simulink model "Voltage_Vector_with_script_fianl"  (R2024b)
settings: Solver=FixedStepAuto  StartTime=0.0  StopTime=0.5  FixedStep=1e-5  RelTol=1e-3
model workspace (MAT data in the model file):
  Cap = 0.004
  FL = 0.025
  Indcut = 0.005
  Initial_Voltage = 125
  R_Load = 1000
  V_dc = 300
  Vd = 125
  Vl = 400
  c = 125
  cap = 7.07e-05
  f_o = 50
  f_s = 5000
libraries: spsIGBTDiodeLib x72, spsSeriesRLCBranchLib x48, spsMultimeterLib x9, spsRMSLib x7, spsThreePhaseBreakerLib x6, spsTHDLib x6, spsThreePhaseSeriesRLCLoadLib x4, spsGroundLib x3, spsCurrentMeasurementLib x2, spsDCVoltageSourceLib x2, spsThreePhaseVIMeasurementLib x2, slpidlib x1
(part 1 of 3)
settings Model: Creator=Ravinga  LastModifiedBy=Sampa
settings DataIOCC: ReturnWorkspaceOutputs=off

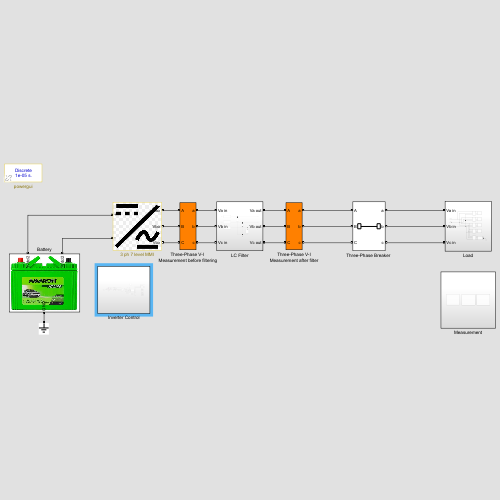
[thumbnail: Simulink's stored preview of the top-level diagram]
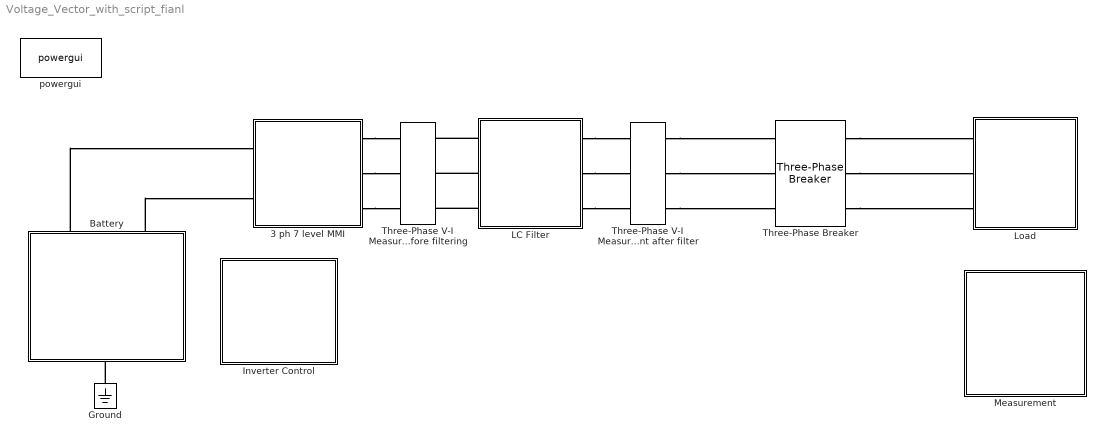
== system Voltage_Vector_with_script_fianl ==
  3 ph 7 level MMI : Subsystem
      mask Display: image('$imagefile'); % Use "Edit Image" on toolstrip to change.
  Battery : Subsystem
      settings: PortSchema="{\"entries\":[{\"content\":{\"sides\":[{\"content\":{},\"type\":\"ConnectorPlacement.EquallySpacedRectSide\",\"uuid\":\"8b3d1574-355a-4c35-8c5c-de7b51b3cb30\"},{\"content\":{\"side\":\"RIGHT\"},\"type\":\"ConnectorPlacement.EquallySpacedRectSide\",\"uuid\":\"59478119-0728-40d5-b667-b9fe531f9ab0\"},{\"content\":{\"connectorIds\":[\"LConn1\",\"LConn2\"],\"side\":\"TOP\"},\"type\":\"ConnectorPlacement.EquallySpacedRectSide\",\"uuid\":\"4590429d-f6cd-431e-b965-edb08c3a41e8\"},{\"content\":{\"connectorIds\":[\"RConn1\"],\"side\":\"BOTTOM\"},\"type\":\"ConnectorPlacement.EquallySpacedRectSide\",\"uuid\":\"66b38a99-a54a-47db-8935-0704255e048e\"}]},\"type\":\"ConnectorPlacement.EquallySpacedConnector\",\"uuid\":\"702254ea-54ff-4f66-b397-10c2b421dddc\"}],\"packageUris\":[\"http://schema.mathworks.com/mf0/Connector/R2020b\"],\"version\":\"1.0\"}"
      mask Display: image('12-v-amaron-battery.jpg');
  Ground : spsGroundLib/Ground  LConnTagsString=a
  Inverter Control : Subsystem
  LC Filter : Subsystem
  Load : Subsystem
  Measurement : Subsystem
  "Three-Phase Breaker " : spsThreePhaseBreakerLib/Three-Phase Breaker  InitialState=closed  SwitchA=on  SwitchB=on  SwitchC=on  SwitchTimes="[1/60  5/60]"  External=off  BreakerResistance=0.01  SnubberResistance=inf  SnubberCapacitance=inf  Measurements=None
  Three-Phase V-I Measurement after filter : spsThreePhaseVIMeasurementLib/Three-Phase V-I Measurement  VoltageMeasurement=phase-to-ground  SetLabelV=on  LabelV=Vabc_af  Vpu=off  VpuLL=off  CurrentMeasurement=yes  SetLabelI=on  LabelI=Iabc_af  Ipu=off  Pbase=100e6  Vbase=500e3  OutputType=Complex  PhasorSimulation=off  PSBequivalent=0
  Three-Phase V-I Measurement before filtering : spsThreePhaseVIMeasurementLib/Three-Phase V-I Measurement  VoltageMeasurement=phase-to-ground  SetLabelV=on  LabelV=Vabc_bf  Vpu=off  VpuLL=off  CurrentMeasurement=yes  SetLabelI=on  LabelI=Iabc_bf  Ipu=off  Pbase=100e6  Vbase=500e3  OutputType=Complex  PhasorSimulation=off  PSBequivalent=0
  powergui : spspowerguiLib/powergui  Priority=1  SimulationMode=Discrete  SampleTime=1e-5  frequency=60  Iterations=50  frequencyindice=0  Pbase=100e6  ErrMax=1e-4  UnitsV=kV  UnitsW=MW  buscounter=0  FunctionMessages=off  echomessages=off  EnableUseOfTLC=off  CurrentSourceSwitches=off  DisableSnubberDevices=off  DisableRonSwitches=off  DisableVfSwitches=off  DisplayEquations=off  AutomaticDiscreteSolvers=off  SolverType=Tustin/Backward Euler (TBE)  Interpol=off  ExternalGateDelay=off  methode=off  Ts=100  x0status=blocks  SPID=on  SwTol=0  HookPort=off  NonlinearTolerance=1e-4  nMaxIteration=100  ContinueOnMaxIteration=off  RestoreLinks=warning  ResistiveCurrentMeasurement=off  Frange=[0:2:500]  Ylog=off  Xlog=on  ShowGrid=off  save=off  variable=ZData  structure=0  ZoomFFT=off  StartTime=0.0  cycles=1  DisplayStyle=1  fundamental=60  FreqAxis=off  MaxFrequency=1000  frequencyindicesteady=1  RmsSteady=1  display=off
  connections:
  3 ph 7 level MMI/RConn1 -- Three-Phase V-I Measurement before filtering/LConn1
  3 ph 7 level MMI/RConn2 -- Three-Phase V-I Measurement before filtering/LConn2
  3 ph 7 level MMI/RConn3 -- Three-Phase V-I Measurement before filtering/LConn3
  "Three-Phase Breaker "/RConn1 -- Load/LConn1
  "Three-Phase Breaker "/RConn2 -- Load/LConn2
  "Three-Phase Breaker "/RConn3 -- Load/LConn3
  LC Filter/LConn1 -- Three-Phase V-I Measurement before filtering/RConn1
  LC Filter/LConn2 -- Three-Phase V-I Measurement before filtering/RConn2
  LC Filter/LConn3 -- Three-Phase V-I Measurement before filtering/RConn3
  LC Filter/RConn1 -- Three-Phase V-I Measurement after filter/LConn1
  LC Filter/RConn2 -- Three-Phase V-I Measurement after filter/LConn2
  LC Filter/RConn3 -- Three-Phase V-I Measurement after filter/LConn3
  Battery/LConn1 -- 3 ph 7 level MMI/LConn1
  Battery/LConn2 -- 3 ph 7 level MMI/LConn2
  Ground/LConn1 -- Battery/RConn1
  Three-Phase V-I Measurement after filter/RConn1 -- "Three-Phase Breaker "/LConn1
  Three-Phase V-I Measurement after filter/RConn2 -- "Three-Phase Breaker "/LConn2
  Three-Phase V-I Measurement after filter/RConn3 -- "Three-Phase Breaker "/LConn3

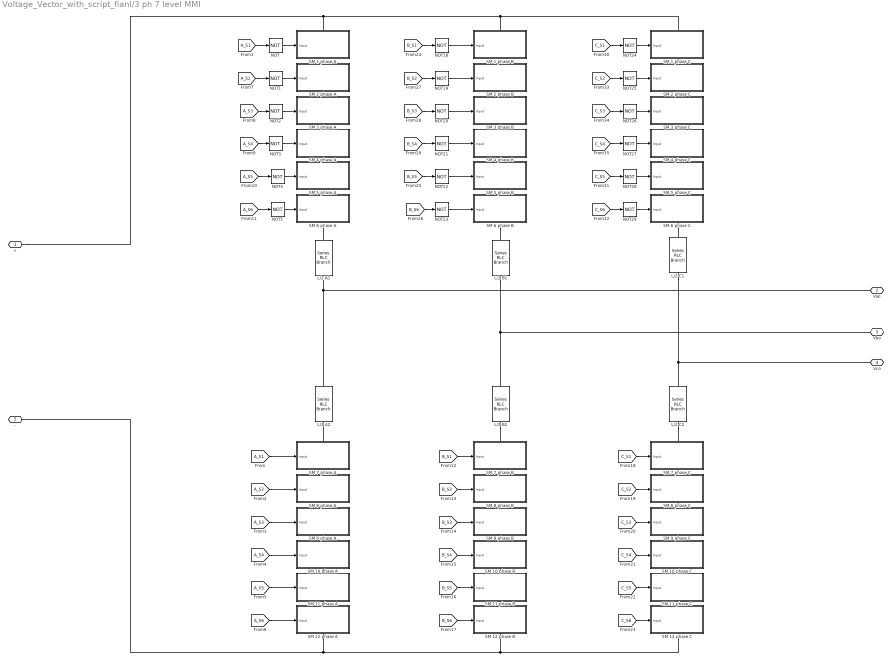
== system Voltage_Vector_with_script_fianl/3 ph 7 level MMI ==
  L/2 A1 : spsSeriesRLCBranchLib/Series RLC Branch  LConnTagsString=__new0  RConnTagsString=__new0  BranchType=L  Resistance=1  Inductance=Indcut  SetiL0=off  InitialCurrent=0  Capacitance=1e-6  Setx0=off  InitialVoltage=0  Measurements=Branch voltage and current
  L/2 A2 : spsSeriesRLCBranchLib/Series RLC Branch  LConnTagsString=__new0  RConnTagsString=__new0  BranchType=L  Resistance=1  Inductance=Indcut  SetiL0=off  InitialCurrent=0  Capacitance=1e-6  Setx0=off  InitialVoltage=0  Measurements=Branch voltage and current
  L/2 B1 : spsSeriesRLCBranchLib/Series RLC Branch  LConnTagsString=__new0  RConnTagsString=__new0  BranchType=L  Resistance=1  Inductance=Indcut  SetiL0=off  InitialCurrent=0  Capacitance=1e-6  Setx0=off  InitialVoltage=0  Measurements=Branch voltage and current
  L/2 B2 : spsSeriesRLCBranchLib/Series RLC Branch  LConnTagsString=__new0  RConnTagsString=__new0  BranchType=L  Resistance=1  Inductance=Indcut  SetiL0=off  InitialCurrent=0  Capacitance=1e-6  Setx0=off  InitialVoltage=0  Measurements=Branch voltage and current
  L/2 C1 : spsSeriesRLCBranchLib/Series RLC Branch  LConnTagsString=__new0  RConnTagsString=__new0  BranchType=L  Resistance=1  Inductance=Indcut  SetiL0=off  InitialCurrent=0  Capacitance=1e-6  Setx0=off  InitialVoltage=0  Measurements=Branch voltage and current
  L/2 C2 : spsSeriesRLCBranchLib/Series RLC Branch  LConnTagsString=__new0  RConnTagsString=__new0  BranchType=L  Resistance=1  Inductance=Indcut  SetiL0=off  InitialCurrent=0  Capacitance=1e-6  Setx0=off  InitialVoltage=0  Measurements=Branch voltage and current
  NOT{,1..5,18..29} (18 alike) : Logic  Operator=NOT  IconShape=distinctive  AllPortsSameDT=off  OutDataTypeStr=boolean
  SM 1 phase A : Subsystem
      settings: PortSchema="{\"entries\":[{\"content\":{\"sides\":[{\"content\":{\"connectorIds\":[\"In1\"]},\"type\":\"ConnectorPlacement.EquallySpacedRectSide\",\"uuid\":\"a2a6df29-5e25-4a5c-b62e-0f1ae4b64f0e\"},{\"content\":{\"connectorIds\":[],\"side\":\"RIGHT\"},\"type\":\"ConnectorPlacement.EquallySpacedRectSide\",\"uuid\":\"30b08227-6494-43ba-ab8b-c0acd0c21381\"},{\"content\":{\"connectorIds\":[\"LConn1\"],\"side\":\"TOP\"},\"type\":\"ConnectorPlacement.EquallySpacedRectSide\",\"uuid\":\"a6e05eb5-068d-4625-ba30-3a309ab3e04e\"},{\"content\":{\"connectorIds\":[\"RConn1\"],\"side\":\"BOTTOM\"},\"type\":\"ConnectorPlacement.EquallySpacedRectSide\",\"uuid\":\"593874a1-6541-4ba7-a8c9-20c2ddfecffb\"}]},\"type\":\"ConnectorPlacement.EquallySpacedConnector\",\"uuid\":\"7a0dd57a-dc4f-41ff-a1a4-3a20e1ff1320\"}],\"packageUris\":[\"http://schema.mathworks.com/mf0/Connector/R2020b\"],\"version\":\"1.0\"}"
  SM 1 phase B : Subsystem
      settings: PortSchema="{\"entries\":[{\"content\":{\"sides\":[{\"content\":{\"connectorIds\":[\"In1\"]},\"type\":\"ConnectorPlacement.EquallySpacedRectSide\",\"uuid\":\"a2a6df29-5e25-4a5c-b62e-0f1ae4b64f0e\"},{\"content\":{\"connectorIds\":[],\"side\":\"RIGHT\"},\"type\":\"ConnectorPlacement.EquallySpacedRectSide\",\"uuid\":\"30b08227-6494-43ba-ab8b-c0acd0c21381\"},{\"content\":{\"connectorIds\":[\"LConn1\"],\"side\":\"TOP\"},\"type\":\"ConnectorPlacement.EquallySpacedRectSide\",\"uuid\":\"a6e05eb5-068d-4625-ba30-3a309ab3e04e\"},{\"content\":{\"connectorIds\":[\"RConn1\"],\"side\":\"BOTTOM\"},\"type\":\"ConnectorPlacement.EquallySpacedRectSide\",\"uuid\":\"593874a1-6541-4ba7-a8c9-20c2ddfecffb\"}]},\"type\":\"ConnectorPlacement.EquallySpacedConnector\",\"uuid\":\"7a0dd57a-dc4f-41ff-a1a4-3a20e1ff1320\"}],\"packageUris\":[\"http://schema.mathworks.com/mf0/Connector/R2020b\"],\"version\":\"1.0\"}"
  SM 1 phase C : Subsystem
      settings: PortSchema="{\"entries\":[{\"content\":{\"sides\":[{\"content\":{\"connectorIds\":[\"In1\"]},\"type\":\"ConnectorPlacement.EquallySpacedRectSide\",\"uuid\":\"a2a6df29-5e25-4a5c-b62e-0f1ae4b64f0e\"},{\"content\":{\"connectorIds\":[],\"side\":\"RIGHT\"},\"type\":\"ConnectorPlacement.EquallySpacedRectSide\",\"uuid\":\"30b08227-6494-43ba-ab8b-c0acd0c21381\"},{\"content\":{\"connectorIds\":[\"LConn1\"],\"side\":\"TOP\"},\"type\":\"ConnectorPlacement.EquallySpacedRectSide\",\"uuid\":\"a6e05eb5-068d-4625-ba30-3a309ab3e04e\"},{\"content\":{\"connectorIds\":[\"RConn1\"],\"side\":\"BOTTOM\"},\"type\":\"ConnectorPlacement.EquallySpacedRectSide\",\"uuid\":\"593874a1-6541-4ba7-a8c9-20c2ddfecffb\"}]},\"type\":\"ConnectorPlacement.EquallySpacedConnector\",\"uuid\":\"7a0dd57a-dc4f-41ff-a1a4-3a20e1ff1320\"}],\"packageUris\":[\"http://schema.mathworks.com/mf0/Connector/R2020b\"],\"version\":\"1.0\"}"
  SM 10 phase A : Subsystem
      settings: PortSchema="{\"entries\":[{\"content\":{\"sides\":[{\"content\":{\"connectorIds\":[\"In1\"]},\"type\":\"ConnectorPlacement.EquallySpacedRectSide\",\"uuid\":\"a2a6df29-5e25-4a5c-b62e-0f1ae4b64f0e\"},{\"content\":{\"connectorIds\":[],\"side\":\"RIGHT\"},\"type\":\"ConnectorPlacement.EquallySpacedRectSide\",\"uuid\":\"30b08227-6494-43ba-ab8b-c0acd0c21381\"},{\"content\":{\"connectorIds\":[\"LConn1\"],\"side\":\"TOP\"},\"type\":\"ConnectorPlacement.EquallySpacedRectSide\",\"uuid\":\"a6e05eb5-068d-4625-ba30-3a309ab3e04e\"},{\"content\":{\"connectorIds\":[\"RConn1\"],\"side\":\"BOTTOM\"},\"type\":\"ConnectorPlacement.EquallySpacedRectSide\",\"uuid\":\"593874a1-6541-4ba7-a8c9-20c2ddfecffb\"}]},\"type\":\"ConnectorPlacement.EquallySpacedConnector\",\"uuid\":\"7a0dd57a-dc4f-41ff-a1a4-3a20e1ff1320\"}],\"packageUris\":[\"http://schema.mathworks.com/mf0/Connector/R2020b\"],\"version\":\"1.0\"}"
  SM 10 phase B : Subsystem
      settings: PortSchema="{\"entries\":[{\"content\":{\"sides\":[{\"content\":{\"connectorIds\":[\"In1\"]},\"type\":\"ConnectorPlacement.EquallySpacedRectSide\",\"uuid\":\"a2a6df29-5e25-4a5c-b62e-0f1ae4b64f0e\"},{\"content\":{\"connectorIds\":[],\"side\":\"RIGHT\"},\"type\":\"ConnectorPlacement.EquallySpacedRectSide\",\"uuid\":\"30b08227-6494-43ba-ab8b-c0acd0c21381\"},{\"content\":{\"connectorIds\":[\"LConn1\"],\"side\":\"TOP\"},\"type\":\"ConnectorPlacement.EquallySpacedRectSide\",\"uuid\":\"a6e05eb5-068d-4625-ba30-3a309ab3e04e\"},{\"content\":{\"connectorIds\":[\"RConn1\"],\"side\":\"BOTTOM\"},\"type\":\"ConnectorPlacement.EquallySpacedRectSide\",\"uuid\":\"593874a1-6541-4ba7-a8c9-20c2ddfecffb\"}]},\"type\":\"ConnectorPlacement.EquallySpacedConnector\",\"uuid\":\"7a0dd57a-dc4f-41ff-a1a4-3a20e1ff1320\"}],\"packageUris\":[\"http://schema.mathworks.com/mf0/Connector/R2020b\"],\"version\":\"1.0\"}"
  SM 10 phase C : Subsystem
      settings: PortSchema="{\"entries\":[{\"content\":{\"sides\":[{\"content\":{\"connectorIds\":[\"In1\"]},\"type\":\"ConnectorPlacement.EquallySpacedRectSide\",\"uuid\":\"a2a6df29-5e25-4a5c-b62e-0f1ae4b64f0e\"},{\"content\":{\"connectorIds\":[],\"side\":\"RIGHT\"},\"type\":\"ConnectorPlacement.EquallySpacedRectSide\",\"uuid\":\"30b08227-6494-43ba-ab8b-c0acd0c21381\"},{\"content\":{\"connectorIds\":[\"LConn1\"],\"side\":\"TOP\"},\"type\":\"ConnectorPlacement.EquallySpacedRectSide\",\"uuid\":\"a6e05eb5-068d-4625-ba30-3a309ab3e04e\"},{\"content\":{\"connectorIds\":[\"RConn1\"],\"side\":\"BOTTOM\"},\"type\":\"ConnectorPlacement.EquallySpacedRectSide\",\"uuid\":\"593874a1-6541-4ba7-a8c9-20c2ddfecffb\"}]},\"type\":\"ConnectorPlacement.EquallySpacedConnector\",\"uuid\":\"7a0dd57a-dc4f-41ff-a1a4-3a20e1ff1320\"}],\"packageUris\":[\"http://schema.mathworks.com/mf0/Connector/R2020b\"],\"version\":\"1.0\"}"
  SM 11 phase A : Subsystem
      settings: PortSchema="{\"entries\":[{\"content\":{\"sides\":[{\"content\":{\"connectorIds\":[\"In1\"]},\"type\":\"ConnectorPlacement.EquallySpacedRectSide\",\"uuid\":\"a2a6df29-5e25-4a5c-b62e-0f1ae4b64f0e\"},{\"content\":{\"connectorIds\":[],\"side\":\"RIGHT\"},\"type\":\"ConnectorPlacement.EquallySpacedRectSide\",\"uuid\":\"30b08227-6494-43ba-ab8b-c0acd0c21381\"},{\"content\":{\"connectorIds\":[\"LConn1\"],\"side\":\"TOP\"},\"type\":\"ConnectorPlacement.EquallySpacedRectSide\",\"uuid\":\"a6e05eb5-068d-4625-ba30-3a309ab3e04e\"},{\"content\":{\"connectorIds\":[\"RConn1\"],\"side\":\"BOTTOM\"},\"type\":\"ConnectorPlacement.EquallySpacedRectSide\",\"uuid\":\"593874a1-6541-4ba7-a8c9-20c2ddfecffb\"}]},\"type\":\"ConnectorPlacement.EquallySpacedConnector\",\"uuid\":\"7a0dd57a-dc4f-41ff-a1a4-3a20e1ff1320\"}],\"packageUris\":[\"http://schema.mathworks.com/mf0/Connector/R2020b\"],\"version\":\"1.0\"}"
  SM 11 phase B : Subsystem
      settings: PortSchema="{\"entries\":[{\"content\":{\"sides\":[{\"content\":{\"connectorIds\":[\"In1\"]},\"type\":\"ConnectorPlacement.EquallySpacedRectSide\",\"uuid\":\"a2a6df29-5e25-4a5c-b62e-0f1ae4b64f0e\"},{\"content\":{\"connectorIds\":[],\"side\":\"RIGHT\"},\"type\":\"ConnectorPlacement.EquallySpacedRectSide\",\"uuid\":\"30b08227-6494-43ba-ab8b-c0acd0c21381\"},{\"content\":{\"connectorIds\":[\"LConn1\"],\"side\":\"TOP\"},\"type\":\"ConnectorPlacement.EquallySpacedRectSide\",\"uuid\":\"a6e05eb5-068d-4625-ba30-3a309ab3e04e\"},{\"content\":{\"connectorIds\":[\"RConn1\"],\"side\":\"BOTTOM\"},\"type\":\"ConnectorPlacement.EquallySpacedRectSide\",\"uuid\":\"593874a1-6541-4ba7-a8c9-20c2ddfecffb\"}]},\"type\":\"ConnectorPlacement.EquallySpacedConnector\",\"uuid\":\"7a0dd57a-dc4f-41ff-a1a4-3a20e1ff1320\"}],\"packageUris\":[\"http://schema.mathworks.com/mf0/Connector/R2020b\"],\"version\":\"1.0\"}"
  SM 11 phase C : Subsystem
      settings: PortSchema="{\"entries\":[{\"content\":{\"sides\":[{\"content\":{\"connectorIds\":[\"In1\"]},\"type\":\"ConnectorPlacement.EquallySpacedRectSide\",\"uuid\":\"a2a6df29-5e25-4a5c-b62e-0f1ae4b64f0e\"},{\"content\":{\"connectorIds\":[],\"side\":\"RIGHT\"},\"type\":\"ConnectorPlacement.EquallySpacedRectSide\",\"uuid\":\"30b08227-6494-43ba-ab8b-c0acd0c21381\"},{\"content\":{\"connectorIds\":[\"LConn1\"],\"side\":\"TOP\"},\"type\":\"ConnectorPlacement.EquallySpacedRectSide\",\"uuid\":\"a6e05eb5-068d-4625-ba30-3a309ab3e04e\"},{\"content\":{\"connectorIds\":[\"RConn1\"],\"side\":\"BOTTOM\"},\"type\":\"ConnectorPlacement.EquallySpacedRectSide\",\"uuid\":\"593874a1-6541-4ba7-a8c9-20c2ddfecffb\"}]},\"type\":\"ConnectorPlacement.EquallySpacedConnector\",\"uuid\":\"7a0dd57a-dc4f-41ff-a1a4-3a20e1ff1320\"}],\"packageUris\":[\"http://schema.mathworks.com/mf0/Connector/R2020b\"],\"version\":\"1.0\"}"
  SM 12 phase A : Subsystem
      settings: PortSchema="{\"entries\":[{\"content\":{\"sides\":[{\"content\":{\"connectorIds\":[\"In1\"]},\"type\":\"ConnectorPlacement.EquallySpacedRectSide\",\"uuid\":\"a2a6df29-5e25-4a5c-b62e-0f1ae4b64f0e\"},{\"content\":{\"connectorIds\":[],\"side\":\"RIGHT\"},\"type\":\"ConnectorPlacement.EquallySpacedRectSide\",\"uuid\":\"30b08227-6494-43ba-ab8b-c0acd0c21381\"},{\"content\":{\"connectorIds\":[\"LConn1\"],\"side\":\"TOP\"},\"type\":\"ConnectorPlacement.EquallySpacedRectSide\",\"uuid\":\"a6e05eb5-068d-4625-ba30-3a309ab3e04e\"},{\"content\":{\"connectorIds\":[\"RConn1\"],\"side\":\"BOTTOM\"},\"type\":\"ConnectorPlacement.EquallySpacedRectSide\",\"uuid\":\"593874a1-6541-4ba7-a8c9-20c2ddfecffb\"}]},\"type\":\"ConnectorPlacement.EquallySpacedConnector\",\"uuid\":\"7a0dd57a-dc4f-41ff-a1a4-3a20e1ff1320\"}],\"packageUris\":[\"http://schema.mathworks.com/mf0/Connector/R2020b\"],\"version\":\"1.0\"}"
  SM 12 phase B : Subsystem
      settings: PortSchema="{\"entries\":[{\"content\":{\"sides\":[{\"content\":{\"connectorIds\":[\"In1\"]},\"type\":\"ConnectorPlacement.EquallySpacedRectSide\",\"uuid\":\"a2a6df29-5e25-4a5c-b62e-0f1ae4b64f0e\"},{\"content\":{\"connectorIds\":[],\"side\":\"RIGHT\"},\"type\":\"ConnectorPlacement.EquallySpacedRectSide\",\"uuid\":\"30b08227-6494-43ba-ab8b-c0acd0c21381\"},{\"content\":{\"connectorIds\":[\"LConn1\"],\"side\":\"TOP\"},\"type\":\"ConnectorPlacement.EquallySpacedRectSide\",\"uuid\":\"a6e05eb5-068d-4625-ba30-3a309ab3e04e\"},{\"content\":{\"connectorIds\":[\"RConn1\"],\"side\":\"BOTTOM\"},\"type\":\"ConnectorPlacement.EquallySpacedRectSide\",\"uuid\":\"593874a1-6541-4ba7-a8c9-20c2ddfecffb\"}]},\"type\":\"ConnectorPlacement.EquallySpacedConnector\",\"uuid\":\"7a0dd57a-dc4f-41ff-a1a4-3a20e1ff1320\"}],\"packageUris\":[\"http://schema.mathworks.com/mf0/Connector/R2020b\"],\"version\":\"1.0\"}"
  SM 12 phase C : Subsystem
      settings: PortSchema="{\"entries\":[{\"content\":{\"sides\":[{\"content\":{\"connectorIds\":[\"In1\"]},\"type\":\"ConnectorPlacement.EquallySpacedRectSide\",\"uuid\":\"a2a6df29-5e25-4a5c-b62e-0f1ae4b64f0e\"},{\"content\":{\"connectorIds\":[],\"side\":\"RIGHT\"},\"type\":\"ConnectorPlacement.EquallySpacedRectSide\",\"uuid\":\"30b08227-6494-43ba-ab8b-c0acd0c21381\"},{\"content\":{\"connectorIds\":[\"LConn1\"],\"side\":\"TOP\"},\"type\":\"ConnectorPlacement.EquallySpacedRectSide\",\"uuid\":\"a6e05eb5-068d-4625-ba30-3a309ab3e04e\"},{\"content\":{\"connectorIds\":[\"RConn1\"],\"side\":\"BOTTOM\"},\"type\":\"ConnectorPlacement.EquallySpacedRectSide\",\"uuid\":\"593874a1-6541-4ba7-a8c9-20c2ddfecffb\"}]},\"type\":\"ConnectorPlacement.EquallySpacedConnector\",\"uuid\":\"7a0dd57a-dc4f-41ff-a1a4-3a20e1ff1320\"}],\"packageUris\":[\"http://schema.mathworks.com/mf0/Connector/R2020b\"],\"version\":\"1.0\"}"
  SM 2 phase A : Subsystem
      settings: PortSchema="{\"entries\":[{\"content\":{\"sides\":[{\"content\":{\"connectorIds\":[\"In1\"]},\"type\":\"ConnectorPlacement.EquallySpacedRectSide\",\"uuid\":\"a2a6df29-5e25-4a5c-b62e-0f1ae4b64f0e\"},{\"content\":{\"connectorIds\":[],\"side\":\"RIGHT\"},\"type\":\"ConnectorPlacement.EquallySpacedRectSide\",\"uuid\":\"30b08227-6494-43ba-ab8b-c0acd0c21381\"},{\"content\":{\"connectorIds\":[\"LConn1\"],\"side\":\"TOP\"},\"type\":\"ConnectorPlacement.EquallySpacedRectSide\",\"uuid\":\"a6e05eb5-068d-4625-ba30-3a309ab3e04e\"},{\"content\":{\"connectorIds\":[\"RConn1\"],\"side\":\"BOTTOM\"},\"type\":\"ConnectorPlacement.EquallySpacedRectSide\",\"uuid\":\"593874a1-6541-4ba7-a8c9-20c2ddfecffb\"}]},\"type\":\"ConnectorPlacement.EquallySpacedConnector\",\"uuid\":\"7a0dd57a-dc4f-41ff-a1a4-3a20e1ff1320\"}],\"packageUris\":[\"http://schema.mathworks.com/mf0/Connector/R2020b\"],\"version\":\"1.0\"}"
  SM 2 phase B : Subsystem
      settings: PortSchema="{\"entries\":[{\"content\":{\"sides\":[{\"content\":{\"connectorIds\":[\"In1\"]},\"type\":\"ConnectorPlacement.EquallySpacedRectSide\",\"uuid\":\"a2a6df29-5e25-4a5c-b62e-0f1ae4b64f0e\"},{\"content\":{\"connectorIds\":[],\"side\":\"RIGHT\"},\"type\":\"ConnectorPlacement.EquallySpacedRectSide\",\"uuid\":\"30b08227-6494-43ba-ab8b-c0acd0c21381\"},{\"content\":{\"connectorIds\":[\"LConn1\"],\"side\":\"TOP\"},\"type\":\"ConnectorPlacement.EquallySpacedRectSide\",\"uuid\":\"a6e05eb5-068d-4625-ba30-3a309ab3e04e\"},{\"content\":{\"connectorIds\":[\"RConn1\"],\"side\":\"BOTTOM\"},\"type\":\"ConnectorPlacement.EquallySpacedRectSide\",\"uuid\":\"593874a1-6541-4ba7-a8c9-20c2ddfecffb\"}]},\"type\":\"ConnectorPlacement.EquallySpacedConnector\",\"uuid\":\"7a0dd57a-dc4f-41ff-a1a4-3a20e1ff1320\"}],\"packageUris\":[\"http://schema.mathworks.com/mf0/Connector/R2020b\"],\"version\":\"1.0\"}"
  SM 2 phase C : Subsystem
      settings: PortSchema="{\"entries\":[{\"content\":{\"sides\":[{\"content\":{\"connectorIds\":[\"In1\"]},\"type\":\"ConnectorPlacement.EquallySpacedRectSide\",\"uuid\":\"a2a6df29-5e25-4a5c-b62e-0f1ae4b64f0e\"},{\"content\":{\"connectorIds\":[],\"side\":\"RIGHT\"},\"type\":\"ConnectorPlacement.EquallySpacedRectSide\",\"uuid\":\"30b08227-6494-43ba-ab8b-c0acd0c21381\"},{\"content\":{\"connectorIds\":[\"LConn1\"],\"side\":\"TOP\"},\"type\":\"ConnectorPlacement.EquallySpacedRectSide\",\"uuid\":\"a6e05eb5-068d-4625-ba30-3a309ab3e04e\"},{\"content\":{\"connectorIds\":[\"RConn1\"],\"side\":\"BOTTOM\"},\"type\":\"ConnectorPlacement.EquallySpacedRectSide\",\"uuid\":\"593874a1-6541-4ba7-a8c9-20c2ddfecffb\"}]},\"type\":\"ConnectorPlacement.EquallySpacedConnector\",\"uuid\":\"7a0dd57a-dc4f-41ff-a1a4-3a20e1ff1320\"}],\"packageUris\":[\"http://schema.mathworks.com/mf0/Connector/R2020b\"],\"version\":\"1.0\"}"
  SM 3 phase A : Subsystem
      settings: PortSchema="{\"entries\":[{\"content\":{\"sides\":[{\"content\":{\"connectorIds\":[\"In1\"]},\"type\":\"ConnectorPlacement.EquallySpacedRectSide\",\"uuid\":\"a2a6df29-5e25-4a5c-b62e-0f1ae4b64f0e\"},{\"content\":{\"connectorIds\":[],\"side\":\"RIGHT\"},\"type\":\"ConnectorPlacement.EquallySpacedRectSide\",\"uuid\":\"30b08227-6494-43ba-ab8b-c0acd0c21381\"},{\"content\":{\"connectorIds\":[\"LConn1\"],\"side\":\"TOP\"},\"type\":\"ConnectorPlacement.EquallySpacedRectSide\",\"uuid\":\"a6e05eb5-068d-4625-ba30-3a309ab3e04e\"},{\"content\":{\"connectorIds\":[\"RConn1\"],\"side\":\"BOTTOM\"},\"type\":\"ConnectorPlacement.EquallySpacedRectSide\",\"uuid\":\"593874a1-6541-4ba7-a8c9-20c2ddfecffb\"}]},\"type\":\"ConnectorPlacement.EquallySpacedConnector\",\"uuid\":\"7a0dd57a-dc4f-41ff-a1a4-3a20e1ff1320\"}],\"packageUris\":[\"http://schema.mathworks.com/mf0/Connector/R2020b\"],\"version\":\"1.0\"}"
  SM 3 phase B : Subsystem
      settings: PortSchema="{\"entries\":[{\"content\":{\"sides\":[{\"content\":{\"connectorIds\":[\"In1\"]},\"type\":\"ConnectorPlacement.EquallySpacedRectSide\",\"uuid\":\"a2a6df29-5e25-4a5c-b62e-0f1ae4b64f0e\"},{\"content\":{\"connectorIds\":[],\"side\":\"RIGHT\"},\"type\":\"ConnectorPlacement.EquallySpacedRectSide\",\"uuid\":\"30b08227-6494-43ba-ab8b-c0acd0c21381\"},{\"content\":{\"connectorIds\":[\"LConn1\"],\"side\":\"TOP\"},\"type\":\"ConnectorPlacement.EquallySpacedRectSide\",\"uuid\":\"a6e05eb5-068d-4625-ba30-3a309ab3e04e\"},{\"content\":{\"connectorIds\":[\"RConn1\"],\"side\":\"BOTTOM\"},\"type\":\"ConnectorPlacement.EquallySpacedRectSide\",\"uuid\":\"593874a1-6541-4ba7-a8c9-20c2ddfecffb\"}]},\"type\":\"ConnectorPlacement.EquallySpacedConnector\",\"uuid\":\"7a0dd57a-dc4f-41ff-a1a4-3a20e1ff1320\"}],\"packageUris\":[\"http://schema.mathworks.com/mf0/Connector/R2020b\"],\"version\":\"1.0\"}"
  SM 3 phase C : Subsystem
      settings: PortSchema="{\"entries\":[{\"content\":{\"sides\":[{\"content\":{\"connectorIds\":[\"In1\"]},\"type\":\"ConnectorPlacement.EquallySpacedRectSide\",\"uuid\":\"a2a6df29-5e25-4a5c-b62e-0f1ae4b64f0e\"},{\"content\":{\"connectorIds\":[],\"side\":\"RIGHT\"},\"type\":\"ConnectorPlacement.EquallySpacedRectSide\",\"uuid\":\"30b08227-6494-43ba-ab8b-c0acd0c21381\"},{\"content\":{\"connectorIds\":[\"LConn1\"],\"side\":\"TOP\"},\"type\":\"ConnectorPlacement.EquallySpacedRectSide\",\"uuid\":\"a6e05eb5-068d-4625-ba30-3a309ab3e04e\"},{\"content\":{\"connectorIds\":[\"RConn1\"],\"side\":\"BOTTOM\"},\"type\":\"ConnectorPlacement.EquallySpacedRectSide\",\"uuid\":\"593874a1-6541-4ba7-a8c9-20c2ddfecffb\"}]},\"type\":\"ConnectorPlacement.EquallySpacedConnector\",\"uuid\":\"7a0dd57a-dc4f-41ff-a1a4-3a20e1ff1320\"}],\"packageUris\":[\"http://schema.mathworks.com/mf0/Connector/R2020b\"],\"version\":\"1.0\"}"
  SM 4 phase A : Subsystem
      settings: PortSchema="{\"entries\":[{\"content\":{\"sides\":[{\"content\":{\"connectorIds\":[\"In1\"]},\"type\":\"ConnectorPlacement.EquallySpacedRectSide\",\"uuid\":\"a2a6df29-5e25-4a5c-b62e-0f1ae4b64f0e\"},{\"content\":{\"connectorIds\":[],\"side\":\"RIGHT\"},\"type\":\"ConnectorPlacement.EquallySpacedRectSide\",\"uuid\":\"30b08227-6494-43ba-ab8b-c0acd0c21381\"},{\"content\":{\"connectorIds\":[\"LConn1\"],\"side\":\"TOP\"},\"type\":\"ConnectorPlacement.EquallySpacedRectSide\",\"uuid\":\"a6e05eb5-068d-4625-ba30-3a309ab3e04e\"},{\"content\":{\"connectorIds\":[\"RConn1\"],\"side\":\"BOTTOM\"},\"type\":\"ConnectorPlacement.EquallySpacedRectSide\",\"uuid\":\"593874a1-6541-4ba7-a8c9-20c2ddfecffb\"}]},\"type\":\"ConnectorPlacement.EquallySpacedConnector\",\"uuid\":\"7a0dd57a-dc4f-41ff-a1a4-3a20e1ff1320\"}],\"packageUris\":[\"http://schema.mathworks.com/mf0/Connector/R2020b\"],\"version\":\"1.0\"}"
  SM 4 phase B : Subsystem
      settings: PortSchema="{\"entries\":[{\"content\":{\"sides\":[{\"content\":{\"connectorIds\":[\"In1\"]},\"type\":\"ConnectorPlacement.EquallySpacedRectSide\",\"uuid\":\"a2a6df29-5e25-4a5c-b62e-0f1ae4b64f0e\"},{\"content\":{\"connectorIds\":[],\"side\":\"RIGHT\"},\"type\":\"ConnectorPlacement.EquallySpacedRectSide\",\"uuid\":\"30b08227-6494-43ba-ab8b-c0acd0c21381\"},{\"content\":{\"connectorIds\":[\"LConn1\"],\"side\":\"TOP\"},\"type\":\"ConnectorPlacement.EquallySpacedRectSide\",\"uuid\":\"a6e05eb5-068d-4625-ba30-3a309ab3e04e\"},{\"content\":{\"connectorIds\":[\"RConn1\"],\"side\":\"BOTTOM\"},\"type\":\"ConnectorPlacement.EquallySpacedRectSide\",\"uuid\":\"593874a1-6541-4ba7-a8c9-20c2ddfecffb\"}]},\"type\":\"ConnectorPlacement.EquallySpacedConnector\",\"uuid\":\"7a0dd57a-dc4f-41ff-a1a4-3a20e1ff1320\"}],\"packageUris\":[\"http://schema.mathworks.com/mf0/Connector/R2020b\"],\"version\":\"1.0\"}"
  SM 4 phase C : Subsystem
      settings: PortSchema="{\"entries\":[{\"content\":{\"sides\":[{\"content\":{\"connectorIds\":[\"In1\"]},\"type\":\"ConnectorPlacement.EquallySpacedRectSide\",\"uuid\":\"a2a6df29-5e25-4a5c-b62e-0f1ae4b64f0e\"},{\"content\":{\"connectorIds\":[],\"side\":\"RIGHT\"},\"type\":\"ConnectorPlacement.EquallySpacedRectSide\",\"uuid\":\"30b08227-6494-43ba-ab8b-c0acd0c21381\"},{\"content\":{\"connectorIds\":[\"LConn1\"],\"side\":\"TOP\"},\"type\":\"ConnectorPlacement.EquallySpacedRectSide\",\"uuid\":\"a6e05eb5-068d-4625-ba30-3a309ab3e04e\"},{\"content\":{\"connectorIds\":[\"RConn1\"],\"side\":\"BOTTOM\"},\"type\":\"ConnectorPlacement.EquallySpacedRectSide\",\"uuid\":\"593874a1-6541-4ba7-a8c9-20c2ddfecffb\"}]},\"type\":\"ConnectorPlacement.EquallySpacedConnector\",\"uuid\":\"7a0dd57a-dc4f-41ff-a1a4-3a20e1ff1320\"}],\"packageUris\":[\"http://schema.mathworks.com/mf0/Connector/R2020b\"],\"version\":\"1.0\"}"
  SM 5 phase A : Subsystem
      settings: PortSchema="{\"entries\":[{\"content\":{\"sides\":[{\"content\":{\"connectorIds\":[\"In1\"]},\"type\":\"ConnectorPlacement.EquallySpacedRectSide\",\"uuid\":\"a2a6df29-5e25-4a5c-b62e-0f1ae4b64f0e\"},{\"content\":{\"connectorIds\":[],\"side\":\"RIGHT\"},\"type\":\"ConnectorPlacement.EquallySpacedRectSide\",\"uuid\":\"30b08227-6494-43ba-ab8b-c0acd0c21381\"},{\"content\":{\"connectorIds\":[\"LConn1\"],\"side\":\"TOP\"},\"type\":\"ConnectorPlacement.EquallySpacedRectSide\",\"uuid\":\"a6e05eb5-068d-4625-ba30-3a309ab3e04e\"},{\"content\":{\"connectorIds\":[\"RConn1\"],\"side\":\"BOTTOM\"},\"type\":\"ConnectorPlacement.EquallySpacedRectSide\",\"uuid\":\"593874a1-6541-4ba7-a8c9-20c2ddfecffb\"}]},\"type\":\"ConnectorPlacement.EquallySpacedConnector\",\"uuid\":\"7a0dd57a-dc4f-41ff-a1a4-3a20e1ff1320\"}],\"packageUris\":[\"http://schema.mathworks.com/mf0/Connector/R2020b\"],\"version\":\"1.0\"}"
  SM 5 phase B : Subsystem
      settings: PortSchema="{\"entries\":[{\"content\":{\"sides\":[{\"content\":{\"connectorIds\":[\"In1\"]},\"type\":\"ConnectorPlacement.EquallySpacedRectSide\",\"uuid\":\"a2a6df29-5e25-4a5c-b62e-0f1ae4b64f0e\"},{\"content\":{\"connectorIds\":[],\"side\":\"RIGHT\"},\"type\":\"ConnectorPlacement.EquallySpacedRectSide\",\"uuid\":\"30b08227-6494-43ba-ab8b-c0acd0c21381\"},{\"content\":{\"connectorIds\":[\"LConn1\"],\"side\":\"TOP\"},\"type\":\"ConnectorPlacement.EquallySpacedRectSide\",\"uuid\":\"a6e05eb5-068d-4625-ba30-3a309ab3e04e\"},{\"content\":{\"connectorIds\":[\"RConn1\"],\"side\":\"BOTTOM\"},\"type\":\"ConnectorPlacement.EquallySpacedRectSide\",\"uuid\":\"593874a1-6541-4ba7-a8c9-20c2ddfecffb\"}]},\"type\":\"ConnectorPlacement.EquallySpacedConnector\",\"uuid\":\"7a0dd57a-dc4f-41ff-a1a4-3a20e1ff1320\"}],\"packageUris\":[\"http://schema.mathworks.com/mf0/Connector/R2020b\"],\"version\":\"1.0\"}"
  SM 5 phase C : Subsystem
      settings: PortSchema="{\"entries\":[{\"content\":{\"sides\":[{\"content\":{\"connectorIds\":[\"In1\"]},\"type\":\"ConnectorPlacement.EquallySpacedRectSide\",\"uuid\":\"a2a6df29-5e25-4a5c-b62e-0f1ae4b64f0e\"},{\"content\":{\"connectorIds\":[],\"side\":\"RIGHT\"},\"type\":\"ConnectorPlacement.EquallySpacedRectSide\",\"uuid\":\"30b08227-6494-43ba-ab8b-c0acd0c21381\"},{\"content\":{\"connectorIds\":[\"LConn1\"],\"side\":\"TOP\"},\"type\":\"ConnectorPlacement.EquallySpacedRectSide\",\"uuid\":\"a6e05eb5-068d-4625-ba30-3a309ab3e04e\"},{\"content\":{\"connectorIds\":[\"RConn1\"],\"side\":\"BOTTOM\"},\"type\":\"ConnectorPlacement.EquallySpacedRectSide\",\"uuid\":\"593874a1-6541-4ba7-a8c9-20c2ddfecffb\"}]},\"type\":\"ConnectorPlacement.EquallySpacedConnector\",\"uuid\":\"7a0dd57a-dc4f-41ff-a1a4-3a20e1ff1320\"}],\"packageUris\":[\"http://schema.mathworks.com/mf0/Connector/R2020b\"],\"version\":\"1.0\"}"
  SM 6 phase A : Subsystem
      settings: PortSchema="{\"entries\":[{\"content\":{\"sides\":[{\"content\":{\"connectorIds\":[\"In1\"]},\"type\":\"ConnectorPlacement.EquallySpacedRectSide\",\"uuid\":\"a2a6df29-5e25-4a5c-b62e-0f1ae4b64f0e\"},{\"content\":{\"connectorIds\":[],\"side\":\"RIGHT\"},\"type\":\"ConnectorPlacement.EquallySpacedRectSide\",\"uuid\":\"30b08227-6494-43ba-ab8b-c0acd0c21381\"},{\"content\":{\"connectorIds\":[\"LConn1\"],\"side\":\"TOP\"},\"type\":\"ConnectorPlacement.EquallySpacedRectSide\",\"uuid\":\"a6e05eb5-068d-4625-ba30-3a309ab3e04e\"},{\"content\":{\"connectorIds\":[\"RConn1\"],\"side\":\"BOTTOM\"},\"type\":\"ConnectorPlacement.EquallySpacedRectSide\",\"uuid\":\"593874a1-6541-4ba7-a8c9-20c2ddfecffb\"}]},\"type\":\"ConnectorPlacement.EquallySpacedConnector\",\"uuid\":\"7a0dd57a-dc4f-41ff-a1a4-3a20e1ff1320\"}],\"packageUris\":[\"http://schema.mathworks.com/mf0/Connector/R2020b\"],\"version\":\"1.0\"}"
  SM 6 phase B : Subsystem
      settings: PortSchema="{\"entries\":[{\"content\":{\"sides\":[{\"content\":{\"connectorIds\":[\"In1\"]},\"type\":\"ConnectorPlacement.EquallySpacedRectSide\",\"uuid\":\"a2a6df29-5e25-4a5c-b62e-0f1ae4b64f0e\"},{\"content\":{\"connectorIds\":[],\"side\":\"RIGHT\"},\"type\":\"ConnectorPlacement.EquallySpacedRectSide\",\"uuid\":\"30b08227-6494-43ba-ab8b-c0acd0c21381\"},{\"content\":{\"connectorIds\":[\"LConn1\"],\"side\":\"TOP\"},\"type\":\"ConnectorPlacement.EquallySpacedRectSide\",\"uuid\":\"a6e05eb5-068d-4625-ba30-3a309ab3e04e\"},{\"content\":{\"connectorIds\":[\"RConn1\"],\"side\":\"BOTTOM\"},\"type\":\"ConnectorPlacement.EquallySpacedRectSide\",\"uuid\":\"593874a1-6541-4ba7-a8c9-20c2ddfecffb\"}]},\"type\":\"ConnectorPlacement.EquallySpacedConnector\",\"uuid\":\"7a0dd57a-dc4f-41ff-a1a4-3a20e1ff1320\"}],\"packageUris\":[\"http://schema.mathworks.com/mf0/Connector/R2020b\"],\"version\":\"1.0\"}"
  SM 6 phase C : Subsystem
      settings: PortSchema="{\"entries\":[{\"content\":{\"sides\":[{\"content\":{\"connectorIds\":[\"In1\"]},\"type\":\"ConnectorPlacement.EquallySpacedRectSide\",\"uuid\":\"a2a6df29-5e25-4a5c-b62e-0f1ae4b64f0e\"},{\"content\":{\"connectorIds\":[],\"side\":\"RIGHT\"},\"type\":\"ConnectorPlacement.EquallySpacedRectSide\",\"uuid\":\"30b08227-6494-43ba-ab8b-c0acd0c21381\"},{\"content\":{\"connectorIds\":[\"LConn1\"],\"side\":\"TOP\"},\"type\":\"ConnectorPlacement.EquallySpacedRectSide\",\"uuid\":\"a6e05eb5-068d-4625-ba30-3a309ab3e04e\"},{\"content\":{\"connectorIds\":[\"RConn1\"],\"side\":\"BOTTOM\"},\"type\":\"ConnectorPlacement.EquallySpacedRectSide\",\"uuid\":\"593874a1-6541-4ba7-a8c9-20c2ddfecffb\"}]},\"type\":\"ConnectorPlacement.EquallySpacedConnector\",\"uuid\":\"7a0dd57a-dc4f-41ff-a1a4-3a20e1ff1320\"}],\"packageUris\":[\"http://schema.mathworks.com/mf0/Connector/R2020b\"],\"version\":\"1.0\"}"
  SM 7 phase A : Subsystem
      settings: PortSchema="{\"entries\":[{\"content\":{\"sides\":[{\"content\":{\"connectorIds\":[\"In1\"]},\"type\":\"ConnectorPlacement.EquallySpacedRectSide\",\"uuid\":\"a2a6df29-5e25-4a5c-b62e-0f1ae4b64f0e\"},{\"content\":{\"connectorIds\":[],\"side\":\"RIGHT\"},\"type\":\"ConnectorPlacement.EquallySpacedRectSide\",\"uuid\":\"30b08227-6494-43ba-ab8b-c0acd0c21381\"},{\"content\":{\"connectorIds\":[\"LConn1\"],\"side\":\"TOP\"},\"type\":\"ConnectorPlacement.EquallySpacedRectSide\",\"uuid\":\"a6e05eb5-068d-4625-ba30-3a309ab3e04e\"},{\"content\":{\"connectorIds\":[\"RConn1\"],\"side\":\"BOTTOM\"},\"type\":\"ConnectorPlacement.EquallySpacedRectSide\",\"uuid\":\"593874a1-6541-4ba7-a8c9-20c2ddfecffb\"}]},\"type\":\"ConnectorPlacement.EquallySpacedConnector\",\"uuid\":\"7a0dd57a-dc4f-41ff-a1a4-3a20e1ff1320\"}],\"packageUris\":[\"http://schema.mathworks.com/mf0/Connector/R2020b\"],\"version\":\"1.0\"}"
  SM 7 phase B : Subsystem
      settings: PortSchema="{\"entries\":[{\"content\":{\"sides\":[{\"content\":{\"connectorIds\":[\"In1\"]},\"type\":\"ConnectorPlacement.EquallySpacedRectSide\",\"uuid\":\"a2a6df29-5e25-4a5c-b62e-0f1ae4b64f0e\"},{\"content\":{\"connectorIds\":[],\"side\":\"RIGHT\"},\"type\":\"ConnectorPlacement.EquallySpacedRectSide\",\"uuid\":\"30b08227-6494-43ba-ab8b-c0acd0c21381\"},{\"content\":{\"connectorIds\":[\"LConn1\"],\"side\":\"TOP\"},\"type\":\"ConnectorPlacement.EquallySpacedRectSide\",\"uuid\":\"a6e05eb5-068d-4625-ba30-3a309ab3e04e\"},{\"content\":{\"connectorIds\":[\"RConn1\"],\"side\":\"BOTTOM\"},\"type\":\"ConnectorPlacement.EquallySpacedRectSide\",\"uuid\":\"593874a1-6541-4ba7-a8c9-20c2ddfecffb\"}]},\"type\":\"ConnectorPlacement.EquallySpacedConnector\",\"uuid\":\"7a0dd57a-dc4f-41ff-a1a4-3a20e1ff1320\"}],\"packageUris\":[\"http://schema.mathworks.com/mf0/Connector/R2020b\"],\"version\":\"1.0\"}"
  SM 7 phase C : Subsystem
      settings: PortSchema="{\"entries\":[{\"content\":{\"sides\":[{\"content\":{\"connectorIds\":[\"In1\"]},\"type\":\"ConnectorPlacement.EquallySpacedRectSide\",\"uuid\":\"a2a6df29-5e25-4a5c-b62e-0f1ae4b64f0e\"},{\"content\":{\"connectorIds\":[],\"side\":\"RIGHT\"},\"type\":\"ConnectorPlacement.EquallySpacedRectSide\",\"uuid\":\"30b08227-6494-43ba-ab8b-c0acd0c21381\"},{\"content\":{\"connectorIds\":[\"LConn1\"],\"side\":\"TOP\"},\"type\":\"ConnectorPlacement.EquallySpacedRectSide\",\"uuid\":\"a6e05eb5-068d-4625-ba30-3a309ab3e04e\"},{\"content\":{\"connectorIds\":[\"RConn1\"],\"side\":\"BOTTOM\"},\"type\":\"ConnectorPlacement.EquallySpacedRectSide\",\"uuid\":\"593874a1-6541-4ba7-a8c9-20c2ddfecffb\"}]},\"type\":\"ConnectorPlacement.EquallySpacedConnector\",\"uuid\":\"7a0dd57a-dc4f-41ff-a1a4-3a20e1ff1320\"}],\"packageUris\":[\"http://schema.mathworks.com/mf0/Connector/R2020b\"],\"version\":\"1.0\"}"
  SM 8 phase A : Subsystem
      settings: PortSchema="{\"entries\":[{\"content\":{\"sides\":[{\"content\":{\"connectorIds\":[\"In1\"]},\"type\":\"ConnectorPlacement.EquallySpacedRectSide\",\"uuid\":\"a2a6df29-5e25-4a5c-b62e-0f1ae4b64f0e\"},{\"content\":{\"connectorIds\":[],\"side\":\"RIGHT\"},\"type\":\"ConnectorPlacement.EquallySpacedRectSide\",\"uuid\":\"30b08227-6494-43ba-ab8b-c0acd0c21381\"},{\"content\":{\"connectorIds\":[\"LConn1\"],\"side\":\"TOP\"},\"type\":\"ConnectorPlacement.EquallySpacedRectSide\",\"uuid\":\"a6e05eb5-068d-4625-ba30-3a309ab3e04e\"},{\"content\":{\"connectorIds\":[\"RConn1\"],\"side\":\"BOTTOM\"},\"type\":\"ConnectorPlacement.EquallySpacedRectSide\",\"uuid\":\"593874a1-6541-4ba7-a8c9-20c2ddfecffb\"}]},\"type\":\"ConnectorPlacement.EquallySpacedConnector\",\"uuid\":\"7a0dd57a-dc4f-41ff-a1a4-3a20e1ff1320\"}],\"packageUris\":[\"http://schema.mathworks.com/mf0/Connector/R2020b\"],\"version\":\"1.0\"}"
  SM 8 phase B : Subsystem
      settings: PortSchema="{\"entries\":[{\"content\":{\"sides\":[{\"content\":{\"connectorIds\":[\"In1\"]},\"type\":\"ConnectorPlacement.EquallySpacedRectSide\",\"uuid\":\"a2a6df29-5e25-4a5c-b62e-0f1ae4b64f0e\"},{\"content\":{\"connectorIds\":[],\"side\":\"RIGHT\"},\"type\":\"ConnectorPlacement.EquallySpacedRectSide\",\"uuid\":\"30b08227-6494-43ba-ab8b-c0acd0c21381\"},{\"content\":{\"connectorIds\":[\"LConn1\"],\"side\":\"TOP\"},\"type\":\"ConnectorPlacement.EquallySpacedRectSide\",\"uuid\":\"a6e05eb5-068d-4625-ba30-3a309ab3e04e\"},{\"content\":{\"connectorIds\":[\"RConn1\"],\"side\":\"BOTTOM\"},\"type\":\"ConnectorPlacement.EquallySpacedRectSide\",\"uuid\":\"593874a1-6541-4ba7-a8c9-20c2ddfecffb\"}]},\"type\":\"ConnectorPlacement.EquallySpacedConnector\",\"uuid\":\"7a0dd57a-dc4f-41ff-a1a4-3a20e1ff1320\"}],\"packageUris\":[\"http://schema.mathworks.com/mf0/Connector/R2020b\"],\"version\":\"1.0\"}"
  SM 8 phase C : Subsystem
      settings: PortSchema="{\"entries\":[{\"content\":{\"sides\":[{\"content\":{\"connectorIds\":[\"In1\"]},\"type\":\"ConnectorPlacement.EquallySpacedRectSide\",\"uuid\":\"a2a6df29-5e25-4a5c-b62e-0f1ae4b64f0e\"},{\"content\":{\"connectorIds\":[],\"side\":\"RIGHT\"},\"type\":\"ConnectorPlacement.EquallySpacedRectSide\",\"uuid\":\"30b08227-6494-43ba-ab8b-c0acd0c21381\"},{\"content\":{\"connectorIds\":[\"LConn1\"],\"side\":\"TOP\"},\"type\":\"ConnectorPlacement.EquallySpacedRectSide\",\"uuid\":\"a6e05eb5-068d-4625-ba30-3a309ab3e04e\"},{\"content\":{\"connectorIds\":[\"RConn1\"],\"side\":\"BOTTOM\"},\"type\":\"ConnectorPlacement.EquallySpacedRectSide\",\"uuid\":\"593874a1-6541-4ba7-a8c9-20c2ddfecffb\"}]},\"type\":\"ConnectorPlacement.EquallySpacedConnector\",\"uuid\":\"7a0dd57a-dc4f-41ff-a1a4-3a20e1ff1320\"}],\"packageUris\":[\"http://schema.mathworks.com/mf0/Connector/R2020b\"],\"version\":\"1.0\"}"
  SM 9 phase A : Subsystem
      settings: PortSchema="{\"entries\":[{\"content\":{\"sides\":[{\"content\":{\"connectorIds\":[\"In1\"]},\"type\":\"ConnectorPlacement.EquallySpacedRectSide\",\"uuid\":\"a2a6df29-5e25-4a5c-b62e-0f1ae4b64f0e\"},{\"content\":{\"connectorIds\":[],\"side\":\"RIGHT\"},\"type\":\"ConnectorPlacement.EquallySpacedRectSide\",\"uuid\":\"30b08227-6494-43ba-ab8b-c0acd0c21381\"},{\"content\":{\"connectorIds\":[\"LConn1\"],\"side\":\"TOP\"},\"type\":\"ConnectorPlacement.EquallySpacedRectSide\",\"uuid\":\"a6e05eb5-068d-4625-ba30-3a309ab3e04e\"},{\"content\":{\"connectorIds\":[\"RConn1\"],\"side\":\"BOTTOM\"},\"type\":\"ConnectorPlacement.EquallySpacedRectSide\",\"uuid\":\"593874a1-6541-4ba7-a8c9-20c2ddfecffb\"}]},\"type\":\"ConnectorPlacement.EquallySpacedConnector\",\"uuid\":\"7a0dd57a-dc4f-41ff-a1a4-3a20e1ff1320\"}],\"packageUris\":[\"http://schema.mathworks.com/mf0/Connector/R2020b\"],\"version\":\"1.0\"}"
  SM 9 phase B : Subsystem
      settings: PortSchema="{\"entries\":[{\"content\":{\"sides\":[{\"content\":{\"connectorIds\":[\"In1\"]},\"type\":\"ConnectorPlacement.EquallySpacedRectSide\",\"uuid\":\"a2a6df29-5e25-4a5c-b62e-0f1ae4b64f0e\"},{\"content\":{\"connectorIds\":[],\"side\":\"RIGHT\"},\"type\":\"ConnectorPlacement.EquallySpacedRectSide\",\"uuid\":\"30b08227-6494-43ba-ab8b-c0acd0c21381\"},{\"content\":{\"connectorIds\":[\"LConn1\"],\"side\":\"TOP\"},\"type\":\"ConnectorPlacement.EquallySpacedRectSide\",\"uuid\":\"a6e05eb5-068d-4625-ba30-3a309ab3e04e\"},{\"content\":{\"connectorIds\":[\"RConn1\"],\"side\":\"BOTTOM\"},\"type\":\"ConnectorPlacement.EquallySpacedRectSide\",\"uuid\":\"593874a1-6541-4ba7-a8c9-20c2ddfecffb\"}]},\"type\":\"ConnectorPlacement.EquallySpacedConnector\",\"uuid\":\"7a0dd57a-dc4f-41ff-a1a4-3a20e1ff1320\"}],\"packageUris\":[\"http://schema.mathworks.com/mf0/Connector/R2020b\"],\"version\":\"1.0\"}"
  SM 9 phase C : Subsystem
      settings: PortSchema="{\"entries\":[{\"content\":{\"sides\":[{\"content\":{\"connectorIds\":[\"In1\"]},\"type\":\"ConnectorPlacement.EquallySpacedRectSide\",\"uuid\":\"a2a6df29-5e25-4a5c-b62e-0f1ae4b64f0e\"},{\"content\":{\"connectorIds\":[],\"side\":\"RIGHT\"},\"type\":\"ConnectorPlacement.EquallySpacedRectSide\",\"uuid\":\"30b08227-6494-43ba-ab8b-c0acd0c21381\"},{\"content\":{\"connectorIds\":[\"LConn1\"],\"side\":\"TOP\"},\"type\":\"ConnectorPlacement.EquallySpacedRectSide\",\"uuid\":\"a6e05eb5-068d-4625-ba30-3a309ab3e04e\"},{\"content\":{\"connectorIds\":[\"RConn1\"],\"side\":\"BOTTOM\"},\"type\":\"ConnectorPlacement.EquallySpacedRectSide\",\"uuid\":\"593874a1-6541-4ba7-a8c9-20c2ddfecffb\"}]},\"type\":\"ConnectorPlacement.EquallySpacedConnector\",\"uuid\":\"7a0dd57a-dc4f-41ff-a1a4-3a20e1ff1320\"}],\"packageUris\":[\"http://schema.mathworks.com/mf0/Connector/R2020b\"],\"version\":\"1.0\"}"
  + : PMIOPort  Side=Left
  Vao : PMIOPort  Port=2  Side=Right
  Vbo : PMIOPort  Port=3  Side=Right
  Vco : PMIOPort  Port=4  Side=Right
  - : PMIOPort  Port=5  Side=Left
  wires:
  [B_S1] -> NOT18/1
  [B_S2] -> NOT19/1
  [B_S3] -> NOT20/1
  [B_S4] -> NOT21/1
  [B_S5] -> NOT22/1
  [B_S6] -> NOT23/1
  [C_S1] -> NOT24/1
  [C_S2] -> NOT25/1
  [C_S3] -> NOT26/1
  [C_S4] -> NOT27/1
  [C_S5] -> NOT28/1
  [C_S6] -> NOT29/1
  [A_S1] -> NOT/1
  [A_S2] -> NOT1/1
  [A_S3] -> NOT2/1
  [A_S5] -> NOT4/1
  [A_S4] -> NOT3/1
  [A_S6] -> NOT5/1
  [B_S1] -> SM 7 phase B/1(Input)
  [B_S2] -> SM 8 phase B/1(Input)
  [B_S3] -> SM 9 phase B/1(Input)
  [B_S4] -> SM 10 phase B/1(Input)
  [B_S5] -> SM 11 phase B/1(Input)
  [B_S6] -> SM 12 phase B/1(Input)
  [C_S1] -> SM 7 phase C/1(Input)
  [C_S2] -> SM 8 phase C/1(Input)
  [C_S3] -> SM 9 phase C/1(Input)
  [C_S4] -> SM 10 phase C/1(Input)
  [C_S5] -> SM 11 phase C/1(Input)
  [C_S6] -> SM 12 phase C/1(Input)
  NOT/1 -> SM 1 phase A/1(Input)
  NOT1/1 -> SM 2 phase A/1(Input)
  NOT2/1 -> SM 3 phase A/1(Input)
  NOT3/1 -> SM 4 phase A/1(Input)
  NOT4/1 -> SM 5 phase A/1(Input)
  NOT5/1 -> SM 6 phase A/1(Input)
  NOT18/1 -> SM 1 phase B/1(Input)
  NOT19/1 -> SM 2 phase B/1(Input)
  NOT20/1 -> SM 3 phase B/1(Input)
  NOT21/1 -> SM 4 phase B/1(Input)
  NOT22/1 -> SM 5 phase B/1(Input)
  NOT23/1 -> SM 6 phase B/1(Input)
  NOT24/1 -> SM 1 phase C/1(Input)
  NOT25/1 -> SM 2 phase C/1(Input)
  NOT26/1 -> SM 3 phase C/1(Input)
  NOT27/1 -> SM 4 phase C/1(Input)
  NOT28/1 -> SM 5 phase C/1(Input)
  NOT29/1 -> SM 6 phase C/1(Input)
  [A_S1] -> SM 7 phase A/1(Input)
  [A_S2] -> SM 8 phase A/1(Input)
  [A_S3] -> SM 9 phase A/1(Input)
  [A_S4] -> SM 10 phase A/1(Input)
  [A_S5] -> SM 11 phase A/1(Input)
  [A_S6] -> SM 12 phase A/1(Input)
  connections:
  SM 3 phase B/RConn1 -- SM 4 phase B/LConn1
  SM 2 phase B/RConn1 -- SM 3 phase B/LConn1
  SM 10 phase B/RConn1 -- SM 11 phase B/LConn1
  L/2 A2/RConn1 -- SM 7 phase A/LConn1
  SM 9 phase C/RConn1 -- SM 10 phase C/LConn1
  SM 9 phase A/RConn1 -- SM 10 phase A/LConn1
  SM 1 phase A/RConn1 -- SM 2 phase A/LConn1
  SM 4 phase A/RConn1 -- SM 5 phase A/LConn1
  SM 11 phase B/RConn1 -- SM 12 phase B/LConn1
  SM 9 phase B/RConn1 -- SM 10 phase B/LConn1
  SM 4 phase C/RConn1 -- SM 5 phase C/LConn1
  SM 6 phase A/RConn1 -- L/2 A1/LConn1
  SM 1 phase B/RConn1 -- SM 2 phase B/LConn1
  L/2 B1/RConn1 -- L/2 B2/LConn1 -- Vbo/RConn1
  SM 12 phase A/RConn1 -- SM 12 phase B/RConn1 -- SM 12 phase C/RConn1 -- -/RConn1
  SM 7 phase A/RConn1 -- SM 8 phase A/LConn1
  SM 8 phase C/RConn1 -- SM 9 phase C/LConn1
  SM 2 phase A/RConn1 -- SM 3 phase A/LConn1
  SM 5 phase A/RConn1 -- SM 6 phase A/LConn1
  SM 6 phase C/RConn1 -- L/2 C1/LConn1
  SM 5 phase B/RConn1 -- SM 6 phase B/LConn1
  SM 3 phase A/RConn1 -- SM 4 phase A/LConn1
  SM 10 phase A/RConn1 -- SM 11 phase A/LConn1
  Vco/RConn1 -- L/2 C2/LConn1 -- L/2 C1/RConn1
  SM 4 phase B/RConn1 -- SM 5 phase B/LConn1
  SM 8 phase A/RConn1 -- SM 9 phase A/LConn1
  SM 8 phase B/RConn1 -- SM 9 phase B/LConn1
  L/2 C2/RConn1 -- SM 7 phase C/LConn1
  SM 11 phase A/RConn1 -- SM 12 phase A/LConn1
  SM 7 phase C/RConn1 -- SM 8 phase C/LConn1
  SM 2 phase C/RConn1 -- SM 3 phase C/LConn1
  SM 10 phase C/RConn1 -- SM 11 phase C/LConn1
  SM 6 phase B/RConn1 -- L/2 B1/LConn1
  L/2 B2/RConn1 -- SM 7 phase B/LConn1
  SM 5 phase C/RConn1 -- SM 6 phase C/LConn1
  SM 1 phase C/RConn1 -- SM 2 phase C/LConn1
  SM 3 phase C/RConn1 -- SM 4 phase C/LConn1
  +/RConn1 -- SM 1 phase A/LConn1 -- SM 1 phase C/LConn1 -- SM 1 phase B/LConn1
  SM 7 phase B/RConn1 -- SM 8 phase B/LConn1
  SM 11 phase C/RConn1 -- SM 12 phase C/LConn1
  L/2 A2/LConn1 -- Vao/RConn1 -- L/2 A1/RConn1

== system Voltage_Vector_with_script_fianl/Battery ==
  Current Measurement : spsCurrentMeasurementLib/Current Measurement  PhasorSimulation=off  OutputType=Complex  PSBequivalent=0
  Current Measurement1 : spsCurrentMeasurementLib/Current Measurement  PhasorSimulation=off  OutputType=Complex  PSBequivalent=0
  DC Voltage Source : spsDCVoltageSourceLib/DC Voltage Source  Amplitude=Vd*3  Measurements=Voltage
  DC Voltage Source1 : spsDCVoltageSourceLib/DC Voltage Source  Amplitude=Vd*3  Measurements=Voltage
  Scope : Scope  NumInputPorts=2
  +Vdc/2 : PMIOPort  Side=Left
  -Vdc/2 : PMIOPort  Port=2  Side=Left
  GND : PMIOPort  Port=3  Side=Right
  tag scope: i_dc_1=global, i_dc_2=global
  wires:
  Current Measurement/1 -> [i_dc_1]
  Current Measurement1/1 -> [i_dc_2]
  [i_dc_2] -> Scope/2
  [i_dc_1] -> Scope/1
  connections:
  Current Measurement/RConn1 -- +Vdc/2/RConn1
  DC Voltage Source1/RConn1 -- GND/RConn1 -- DC Voltage Source/LConn1
  Current Measurement/LConn1 -- DC Voltage Source/RConn1
  DC Voltage Source1/LConn1 -- Current Measurement1/RConn1
  Current Measurement1/LConn1 -- -Vdc/2/RConn1
